simulink model "MAIN_model"  (R2021a)
settings: Solver=VariableStepAuto  StartTime=0.0  StopTime=10.0  RelTol=1e-3
settings Model: Creator=Dimitris  LastModifiedBy=Dimitris

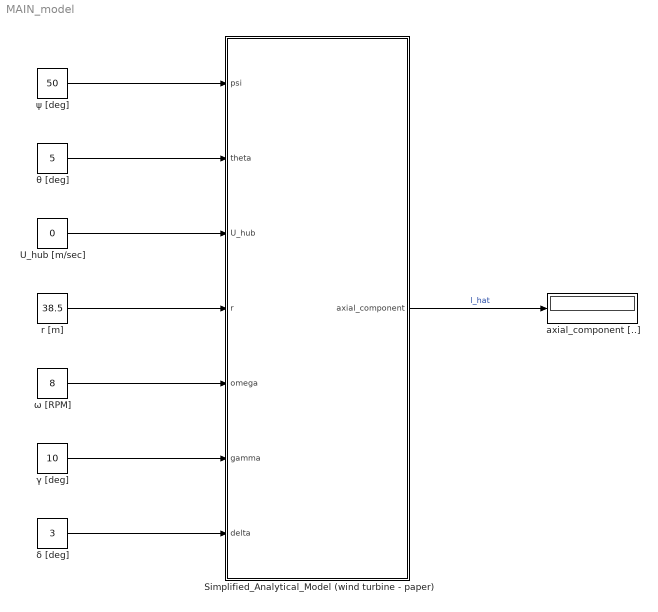
== system MAIN_model ==
  Simplified_Analytical_Model (wind turbine - paper) : Subsystem
  U_hub [m/sec] : Constant  Value=0
  axial_component [..] : Display
  r [m] : Constant  Value=38.5
  γ [deg] : Constant  Value=10
  δ [deg] : Constant  Value=3
  θ [deg] : Constant  Value=5
  ψ [deg] : Constant  Value=50
  ω [RPM] : Constant  Value=8
  wires:
  ψ [deg]/1 -> Simplified_Analytical_Model (wind turbine - paper)/1(psi)
  Simplified_Analytical_Model (wind turbine - paper)/1(axial_component) -> axial_component [..]/1  "l_hat"
  θ [deg]/1 -> Simplified_Analytical_Model (wind turbine - paper)/2(theta)
  U_hub [m/sec]/1 -> Simplified_Analytical_Model (wind turbine - paper)/3(U_hub)
  r [m]/1 -> Simplified_Analytical_Model (wind turbine - paper)/4(r)
  ω [RPM]/1 -> Simplified_Analytical_Model (wind turbine - paper)/5(omega)
  γ [deg]/1 -> Simplified_Analytical_Model (wind turbine - paper)/6(gamma)
  δ [deg]/1 -> Simplified_Analytical_Model (wind turbine - paper)/7(delta)

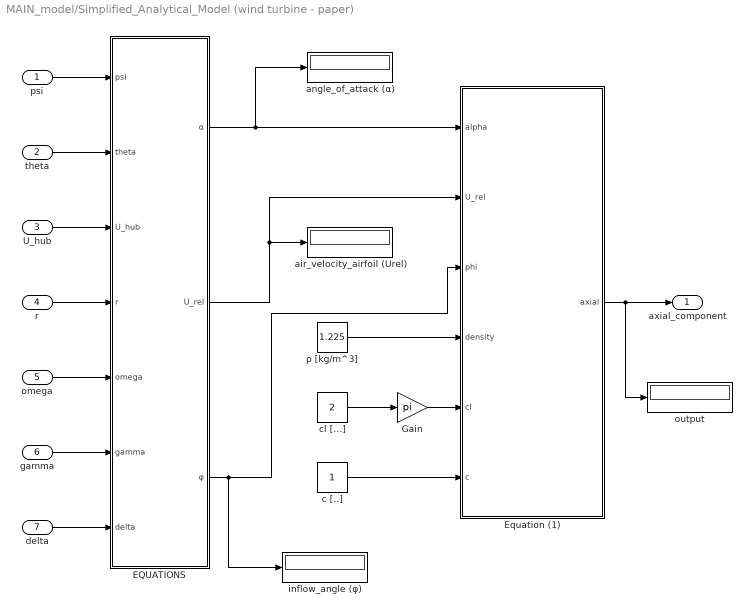
== system MAIN_model/Simplified_Analytical_Model (wind turbine - paper) ==
  psi : Inport
  theta : Inport  Port=2
  U_hub : Inport  Port=3
  r : Inport  Port=4
  omega : Inport  Port=5
  gamma : Inport  Port=6
  delta : Inport  Port=7
  EQUATIONS : Subsystem
  Equation (1) : MATLAB Function  TreatAsAtomicUnit=on
  Gain : Gain  Gain=pi
  air_velocity_airfoil (Urel) : Display
  angle_of_attack (α) : Display
  c [..] : Constant
  cl [...] : Constant  Value=2
  inflow_angle (φ) : Display
  output : Display
  ρ [kg/m^3] : Constant  Value=1.225
  axial_component : Outport
  wires:
  psi/1 -> EQUATIONS/1(psi)
  EQUATIONS/1(α) -> angle_of_attack (α)/1, Equation (1)/1(alpha)
  Equation (1)/1(axial) -> axial_component/1, output/1
  EQUATIONS/2(U_rel) -> Equation (1)/2(U_rel), air_velocity_airfoil (Urel)/1
  EQUATIONS/3(φ) -> inflow_angle (φ)/1, Equation (1)/3(phi)
  ρ [kg/m^3]/1 -> Equation (1)/4(density)
  Gain/1 -> Equation (1)/5(cl)
  cl [...]/1 -> Gain/1
  c [..]/1 -> Equation (1)/6(c)
  theta/1 -> EQUATIONS/2(theta)
  U_hub/1 -> EQUATIONS/3(U_hub)
  r/1 -> EQUATIONS/4(r)
  omega/1 -> EQUATIONS/5(omega)
  gamma/1 -> EQUATIONS/6(gamma)
  delta/1 -> EQUATIONS/7(delta)

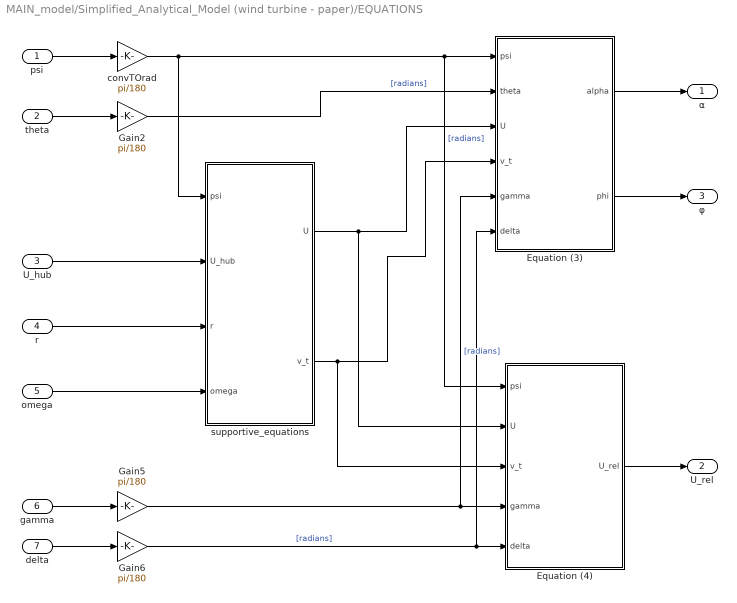
== system MAIN_model/Simplified_Analytical_Model (wind turbine - paper)/EQUATIONS ==
  psi : Inport
  theta : Inport  Port=2
  U_hub : Inport  Port=3
  r : Inport  Port=4
  omega : Inport  Port=5
  gamma : Inport  Port=6
  delta : Inport  Port=7
  Equation (3) : MATLAB Function  TreatAsAtomicUnit=on
  Equation (4) : MATLAB Function  TreatAsAtomicUnit=on
  Gain2 : Gain  Gain=pi/180
  Gain5 : Gain  Gain=pi/180
  Gain6 : Gain  Gain=pi/180
  convTOrad : Gain  Gain=pi/180
  supportive_equations : Subsystem
  α : Outport
  U_rel : Outport  Port=2
  φ : Outport  Port=3
  wires:
  delta/1 -> Gain6/1
  gamma/1 -> Gain5/1
  psi/1 -> convTOrad/1
  theta/1 -> Gain2/1
  convTOrad/1 -> Equation (4)/1(psi), Equation (3)/1(psi), supportive_equations/1(psi)  "[radians]"
  Gain6/1 -> Equation (3)/6(delta), Equation (4)/5(delta)  "[radians]"
  Gain5/1 -> Equation (4)/4(gamma), Equation (3)/5(gamma)  "[radians]"
  Gain2/1 -> Equation (3)/2(theta)  "[radians]"
  Equation (3)/1(alpha) -> α/1
  Equation (3)/2(phi) -> φ/1
  Equation (4)/1(U_rel) -> U_rel/1
  U_hub/1 -> supportive_equations/2(U_hub)
  r/1 -> supportive_equations/3(r)
  omega/1 -> supportive_equations/4(omega)
  supportive_equations/1(U) -> Equation (3)/3(U), Equation (4)/2(U)
  supportive_equations/2(v_t) -> Equation (3)/4(v_t), Equation (4)/3(v_t)

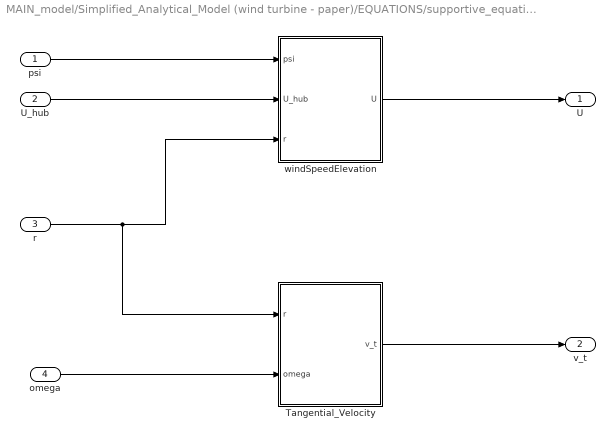
== system MAIN_model/Simplified_Analytical_Model (wind turbine - paper)/EQUATIONS/supportive_equations ==
  psi : Inport
  U_hub : Inport  Port=2
  r : Inport  Port=3
  omega : Inport  Port=4
  Tangential_Velocity : MATLAB Function  TreatAsAtomicUnit=on
  windSpeedElevation : MATLAB Function  TreatAsAtomicUnit=on
  U : Outport
  v_t : Outport  Port=2
  wires:
  Tangential_Velocity/1(v_t) -> v_t/1
  windSpeedElevation/1(U) -> U/1
  psi/1 -> windSpeedElevation/1(psi)
  U_hub/1 -> windSpeedElevation/2(U_hub)
  r/1 -> Tangential_Velocity/1(r), windSpeedElevation/3(r)
  omega/1 -> Tangential_Velocity/2(omega)

== matlab function MAIN_model/Simplified_Analytical_Model (wind turbine - paper)/Equation (1) ==
  data: alpha input; axial output; U_rel input; phi input; density input; cl input; c input
function axial = axialComponent(alpha, U_rel, phi, density, cl, c)
axial = 0.5*density*U_rel^2*cl*alpha*c*cos(phi);

== matlab function MAIN_model/Simplified_Analytical_Model (wind turbine - paper)/EQUATIONS/Equation (3) ==
  data: alpha output; phi output; psi input; theta input; U input; v_t input; gamma input; delta input
function [alpha, phi] = AngleOFAttack(psi, theta, U, v_t, gamma, delta)
phi = atan((U*cos(gamma)*cos(delta)) / ((v_t-U)*(cos(gamma)*sin(delta)*sin(psi) + sin(gamma)*cos(psi))));
alpha = phi - theta;

== matlab function MAIN_model/Simplified_Analytical_Model (wind turbine - paper)/EQUATIONS/Equation (4) ==
  data: U_rel output; psi input; U input; v_t input; gamma input; delta input
function U_rel = airVelocityAirfoil(psi, U, v_t, gamma, delta)
U_rel = sqrt((U*cos(gamma)*cos(delta))^2 + ((v_t-U)*(cos(gamma)*sin(delta)*sin(psi)+(sin(gamma)*cos(psi))))^2);

== matlab function MAIN_model/Simplified_Analytical_Model (wind turbine - paper)/EQUATIONS/supportive_equations/windSpeedElevation ==
  data: psi input; U_hub input; r input; U output
function U = windSpeedElevation(psi, U_hub, r)
U = U_hub + 10; % we need an equation for U that includes psi,r,Uhub

== matlab function MAIN_model/Simplified_Analytical_Model (wind turbine - paper)/EQUATIONS/supportive_equations/Tangential_Velocity ==
  data: r input; omega input; v_t output
function v_t = tangentialVelocity(r, omega)
v_t = omega * r * (2*pi/60);
